simulink model "SEL751Test_Model_1"  (Simulink 8.1)
settings: Solver=ode4  StartTime=0.0  StopTime=inf  FixedStep=Ts  MaxStep=1e-3  RelTol=1e-3
PostLoadFcn:
  | Ts=100e-6; HILLTOP_init;SIM_HIL=1
InitFcn:
  | Ts=100e-6; HILLTOP_init;SIM_HIL=1
values from neighbouring files (symbols this model uses):
  relay_par = xlsread('relay_parameters.xlsx')    [relay_settings_init.m]
undefined symbols (not defined in the file or in its folder): fdesignblkfcn, gcbh, Left, NG_CHP, NG_CHP_lib, ph, type, V
libraries: simulink x23, rtio_opalrt_common x21, rtlab x7, simulink_extras x7, artemis x5, rteventslib x4, Load_lib x3, cables_lib x3, breaker_lib x3, powerlib x2, rtio_generic_modbus x2, transformer_lib x2
(part 2 of 2)

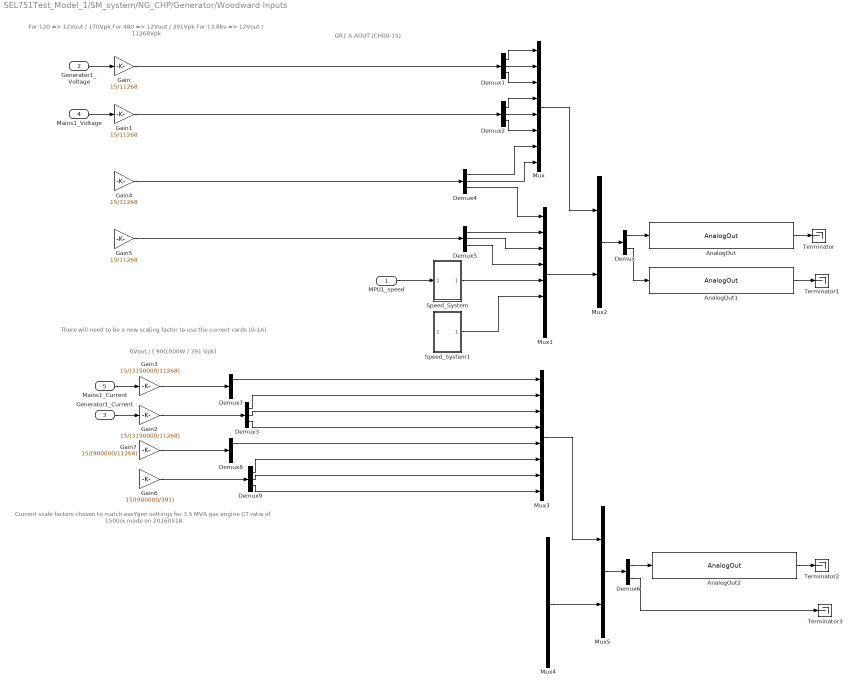
== system SEL751Test_Model_1/SM_system/NG_CHP/Generator/Woodward Inputs ==
  note: There will need to be a
      | new scaling factor to use
      | the current cards (0-1A)
  note: GR1 A AOUT (CH00-15)
  note: For 120 => 12Vout / 170Vpk
      | For 480 => 12Vout / 391Vpk
      | For 13.8kv => 12Vout / 11268Vpk
  note: 6Vout / ( 900,000W / 391 Vpk)
  note: Current scale factors chosen to match
      | easYgen settings for 3.5 MVA gas engine
      | CT ratio of 1500/x made on 20160518
  MPU1_speed : Inport
  Generator1_Voltage : Inport  Port=2
  Generator1_Current : Inport  Port=3
  Mains1_Voltage : Inport  Port=4
  Mains1_Current : Inport  Port=5
  AnalogOut : rtio_opalrt_common/AnalogOut  CtrlName='OpCtrl'  portNb=1  FcnNos=Slot 1 Module A Subsection 1  size=16  maxcount=8  count=8  numchan=8  israngeinput=off  voltagerange=[-16 ... 16]  slot=0  side=0  mismatch=0  slotside=Slot_1_Module_A
      settings: AttributesFormatString=%<CtrlName>
  AnalogOut1 : rtio_opalrt_common/AnalogOut  CtrlName='OpCtrl'  portNb=2  FcnNos=Slot 1 Module A Subsection 2  size=16  maxcount=8  count=8  numchan=8  israngeinput=off  voltagerange=[-16 ... 16]  slot=0  side=0  mismatch=0  slotside=Slot_1_Module_A
      settings: AttributesFormatString=%<CtrlName>
  AnalogOut2 : rtio_opalrt_common/AnalogOut  CtrlName='OpCtrl'  portNb=3  FcnNos=Slot 2 Module A Subsection 1  size=16  maxcount=8  count=8  numchan=8  israngeinput=off  voltagerange=[-16 ... 16]  slot=1  side=0  mismatch=0  slotside=Slot_2_Module_A
      settings: AttributesFormatString=%<CtrlName>
  Demux : Demux  Outputs=2
  Demux{1..5,7..9} (8 alike) : Demux  Outputs=3
  Demux6 : Demux  Outputs=2
  Gain{,1,4..5} (4 alike) : Gain  Gain=15/11268
  Gain2 : Gain  Gain=15/(3150000/11268)
  Gain3 : Gain  Gain=15/(3150000/11268)
  Gain6 : Gain  Gain=15/(900000/391)
  Gain7 : Gain  Gain=15/(900000/11268)
  Mux{,1,3..4} (4 alike) : Mux  Inputs=8
  Mux2 : Mux  Inputs=2
  Mux5 : Mux  Inputs=2
  Speed_System : Subsystem
  Speed_System1 : Subsystem
  Terminator{,1..3} (4 alike) : Terminator
  wires:
  Demux9/3 -> Mux3/8
  Demux9/2 -> Mux3/7
  Demux9/1 -> Mux3/6
  Gain6/1 -> Demux9/1
  Demux8/1 -> Mux3/5
  Gain7/1 -> Demux8/1
  ? -> Gain7/1
  ? -> Gain6/1
  Speed_System1/1(Out1) -> Mux1/6
  ? -> Speed_System1/1(In1)
  ? -> Gain4/1
  ? -> Gain5/1
  Gain4/1 -> Demux4/1
  Gain5/1 -> Demux5/1
  Demux7/1 -> Mux3/1
  Gain3/1 -> Demux7/1
  Mains1_Current/1 -> Gain3/1
  Demux3/3 -> Mux3/4
  Demux3/2 -> Mux3/3
  Demux3/1 -> Mux3/2
  Gain2/1 -> Demux3/1
  AnalogOut2/1 -> Terminator2/1
  Demux6/2 -> Terminator3/1
  Demux6/1 -> AnalogOut2/1
  Mux3/1 -> Mux5/1
  Mux4/1 -> Mux5/2
  Mux5/1 -> Demux6/1
  Demux5/3 -> Mux1/4
  Demux5/2 -> Mux1/3
  Demux5/1 -> Mux1/2
  Demux4/3 -> Mux1/1
  Demux4/2 -> Mux/8
  Demux4/1 -> Mux/7
  Speed_System/1(Out1) -> Mux1/5
  Demux2/3 -> Mux/6
  Demux2/2 -> Mux/5
  Demux2/1 -> Mux/4
  Demux1/3 -> Mux/3
  Demux1/2 -> Mux/2
  Demux1/1 -> Mux/1
  AnalogOut/1 -> Terminator/1
  AnalogOut1/1 -> Terminator1/1
  Demux/1 -> AnalogOut/1
  Demux/2 -> AnalogOut1/1
  Generator1_Voltage/1 -> Gain/1
  Mux/1 -> Mux2/1
  Mux1/1 -> Mux2/2
  Mux2/1 -> Demux/1
  Mains1_Voltage/1 -> Gain1/1
  Gain/1 -> Demux1/1
  Gain1/1 -> Demux2/1
  Generator1_Current/1 -> Gain2/1
  MPU1_speed/1 -> Speed_System/1(In1)

== system SEL751Test_Model_1/SM_system/NG_CHP/Generator/Woodward Outputs ==
  Digital Output : Inport
  DIO Enable : Inport  Port=2
  Bias Enable : Inport  Port=3
  Gen1 MCB Status : Inport  Port=4
  Gen2 MCB Status : Inport  Port=5
  Bus Creator1 : BusCreator  Inputs=3
  DIO - Gr3 : Subsystem
  DIO - Woodward : Subsystem
  DOUT type config : Subsystem
  OpCtrl : rtio_opalrt_common/OpCtrl  CtrlName='OpCtrl'  boardid=0  BitstreamFilename=VC707_2-EX-0001-2_2_6_61-32AIO16DIO16DIOSel-01-01.bin  numconfig=-1  mode=Master  externalClock=off  decimRtsi=0  calibIO=off  SampleTime=0  loadinport=-1  BoardType=VC707  SecondaryPresent=off  sync_type=Audio
  PWM IO - Gr3 : Subsystem
  TSDIO - Gr3 : Subsystem
  Woodward Primary Inputs : Subsystem
  Error : Outport
  IDs : Outport  Port=2
  Digital Inputs : Outport  Port=3
  Gen1 Gov and AVR : Outport  Port=4
  Gen1 Fuel Enable : Outport  Port=5
  Gen1 GCB : Outport  Port=6
  Gen1 MCB : Outport  Port=7
  wires:
  Gen2 MCB Status/1 -> DIO - Woodward/6(Gen2 MCB Status)
  Gen1 MCB Status/1 -> DIO - Woodward/5(Gen1 MCB Status)
  DIO - Woodward/1(Gen1 Fuel Enable) -> Gen1 Fuel Enable/1
  DIO - Woodward/3(Gen1 MCB) -> Gen1 MCB/1
  DIO - Woodward/2(Gen1 GCB) -> Gen1 GCB/1
  Digital Output/1 -> TSDIO - Gr3/1(TSDout), PWM IO - Gr3/1(PWMOut), DIO - Woodward/2(Din_sim)
  Bias Enable/1 -> Woodward Primary Inputs/1(Bias-ctrl)
  Woodward Primary Inputs/1(Gen1 Gov and AVR) -> Gen1 Gov and AVR/1
  DIO Enable/1 -> DIO - Woodward/4(control1), DIO - Woodward/3(control)
  Bus Creator1/1 -> Digital Inputs/1
  DIO - Gr3/1(DIn) -> DIO - Woodward/1(Din_Wood1), Bus Creator1/1  "DIN"
  TSDIO - Gr3/1(TSDin) -> Bus Creator1/2  "TSDIN"
  PWM IO - Gr3/1(PWMIn) -> Bus Creator1/3  "PWMIN"
  DIO - Woodward/4(DIn1) -> DIO - Gr3/1(Dout)
  OpCtrl/2 -> IDs/1
  OpCtrl/1 -> Error/1

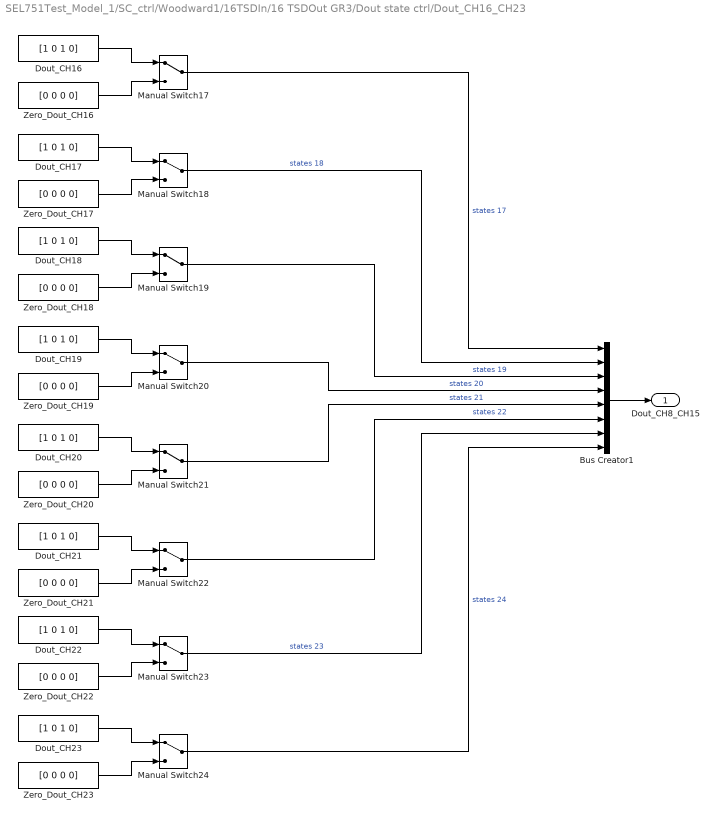
== system SEL751Test_Model_1/SC_ctrl/Woodward1/16TSDIn/16 TSDOut GR3/Dout state ctrl/Dout_CH16_CH23 ==
  Bus Creator1 : BusCreator  Inputs=8
  Dout_CH{16..23} (8 alike) : Constant  Value=[1 0 1 0]
  Manual Switch{17..24} (8 alike) : ManualSwitch
  Zero_Dout_CH{16..23} (8 alike) : Constant  Value=[0 0 0 0]
  Dout_CH8_CH15 : Outport
  wires:
  Bus Creator1/1 -> Dout_CH8_CH15/1
  Dout_CH16/1 -> Manual Switch17/1
  Zero_Dout_CH16/1 -> Manual Switch17/2
  Dout_CH17/1 -> Manual Switch18/1
  Zero_Dout_CH17/1 -> Manual Switch18/2
  Dout_CH18/1 -> Manual Switch19/1
  Zero_Dout_CH18/1 -> Manual Switch19/2
  Dout_CH19/1 -> Manual Switch20/1
  Zero_Dout_CH19/1 -> Manual Switch20/2
  Dout_CH20/1 -> Manual Switch21/1
  Zero_Dout_CH20/1 -> Manual Switch21/2
  Dout_CH21/1 -> Manual Switch22/1
  Zero_Dout_CH21/1 -> Manual Switch22/2
  Dout_CH22/1 -> Manual Switch23/1
  Zero_Dout_CH22/1 -> Manual Switch23/2
  Dout_CH23/1 -> Manual Switch24/1
  Zero_Dout_CH23/1 -> Manual Switch24/2
  Manual Switch17/1 -> Bus Creator1/1  "states 17"
  Manual Switch18/1 -> Bus Creator1/2  "states 18"
  Manual Switch19/1 -> Bus Creator1/3  "states 19"
  Manual Switch20/1 -> Bus Creator1/4  "states 20"
  Manual Switch21/1 -> Bus Creator1/5  "states 21"
  Manual Switch22/1 -> Bus Creator1/6  "states 22"
  Manual Switch23/1 -> Bus Creator1/7  "states 23"
  Manual Switch24/1 -> Bus Creator1/8  "states 24"

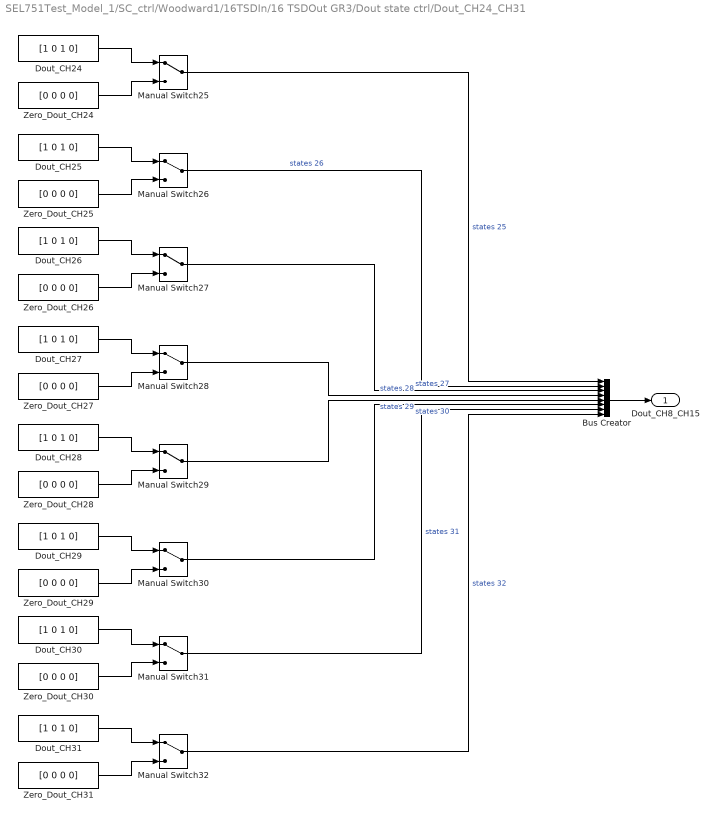
== system SEL751Test_Model_1/SC_ctrl/Woodward1/16TSDIn/16 TSDOut GR3/Dout state ctrl/Dout_CH24_CH31 ==
  Bus Creator : BusCreator  Inputs=8
  Dout_CH{24..31} (8 alike) : Constant  Value=[1 0 1 0]
  Manual Switch{25..32} (8 alike) : ManualSwitch
  Zero_Dout_CH{24..31} (8 alike) : Constant  Value=[0 0 0 0]
  Dout_CH8_CH15 : Outport
  wires:
  Manual Switch32/1 -> Bus Creator/8  "states 32"
  Manual Switch31/1 -> Bus Creator/7  "states 31"
  Manual Switch30/1 -> Bus Creator/6  "states 30"
  Manual Switch29/1 -> Bus Creator/5  "states 29"
  Manual Switch28/1 -> Bus Creator/4  "states 28"
  Manual Switch27/1 -> Bus Creator/3  "states 27"
  Manual Switch26/1 -> Bus Creator/2  "states 26"
  Manual Switch25/1 -> Bus Creator/1  "states 25"
  Zero_Dout_CH31/1 -> Manual Switch32/2
  Dout_CH31/1 -> Manual Switch32/1
  Zero_Dout_CH30/1 -> Manual Switch31/2
  Dout_CH30/1 -> Manual Switch31/1
  Zero_Dout_CH29/1 -> Manual Switch30/2
  Dout_CH29/1 -> Manual Switch30/1
  Zero_Dout_CH28/1 -> Manual Switch29/2
  Dout_CH28/1 -> Manual Switch29/1
  Zero_Dout_CH27/1 -> Manual Switch28/2
  Dout_CH27/1 -> Manual Switch28/1
  Zero_Dout_CH26/1 -> Manual Switch27/2
  Dout_CH26/1 -> Manual Switch27/1
  Zero_Dout_CH25/1 -> Manual Switch26/2
  Dout_CH25/1 -> Manual Switch26/1
  Zero_Dout_CH24/1 -> Manual Switch25/2
  Dout_CH24/1 -> Manual Switch25/1
  Bus Creator/1 -> Dout_CH8_CH15/1

== system SEL751Test_Model_1/SM_system/NG_CHP/Generator/Woodward Inputs/Speed_System ==
  In1 : Inport
  Clock1 : Clock
      settings: DisableCoverage=on
  Duty : Constant  DisableCoverage=on  Value=0.5
  Gain1 : Gain  Gain=5
  Gain3 : Gain  Gain=5
  Gain4 : Gain  Gain=1800
  Output : Trigonometry
  Product1 : Product  DisableCoverage=on  SaturateOnIntegerOverflow=on  InputSameDT=on  OutDataTypeStr=Inherit: Same as first input
  Product3 : Product  DisableCoverage=on  SaturateOnIntegerOverflow=on  InputSameDT=on  OutDataTypeStr=Inherit: Same as first input
  RTE Conversion : rteventslib/Signal Attributes/RTE Conversion  inputdatatype=RTE Boolean  outputdatatype=Double  compensation=Disabled  nbMaxEvents=10  sampleTime=Ts
  RTE SPWM : rteventslib/Sources/RTE SPWM  NumberPhases=1-ph  CenterAlignmentMode=On  MaxFreq=inf  MinFreq=0  EnablingPort=off  ComplementaryMode=off  SpaceVector=off  RiseTimeDelay=0  MaxEvents=10  SampleTime=Ts
  initialFreq : Constant  DisableCoverage=on  Value=2*pi
  Out1 : Outport
  wires:
  Product1/1 -> Output/1
  Clock1/1 -> Product1/1
  initialFreq/1 -> Product3/1
  Product3/1 -> Product1/2
  Gain4/1 -> Product3/2, RTE SPWM/1
  Output/1 -> Gain3/1
  In1/1 -> Gain4/1
  RTE SPWM/1 -> RTE Conversion/1
  Duty/1 -> RTE SPWM/2
  RTE Conversion/1 -> Gain1/1
  Gain1/1 -> Out1/1

== system SEL751Test_Model_1/SM_system/NG_CHP/Generator/Woodward Inputs/Speed_System1 ==
  In1 : Inport
  Clock1 : Clock
      settings: DisableCoverage=on
  Duty : Constant  DisableCoverage=on  Value=0.5
  Gain1 : Gain  Gain=5
  Gain3 : Gain  Gain=5
  Gain4 : Gain  Gain=1800
  Output : Trigonometry
  Product1 : Product  DisableCoverage=on  SaturateOnIntegerOverflow=on  InputSameDT=on  OutDataTypeStr=Inherit: Same as first input
  Product3 : Product  DisableCoverage=on  SaturateOnIntegerOverflow=on  InputSameDT=on  OutDataTypeStr=Inherit: Same as first input
  RTE Conversion : rteventslib/Signal Attributes/RTE Conversion  inputdatatype=RTE Boolean  outputdatatype=Double  compensation=Disabled  nbMaxEvents=10  sampleTime=Ts
  RTE SPWM : rteventslib/Sources/RTE SPWM  NumberPhases=1-ph  CenterAlignmentMode=On  MaxFreq=inf  MinFreq=0  EnablingPort=off  ComplementaryMode=off  SpaceVector=off  RiseTimeDelay=0  MaxEvents=10  SampleTime=Ts
  initialFreq : Constant  DisableCoverage=on  Value=2*pi
  Out1 : Outport
  wires:
  Product1/1 -> Output/1
  Clock1/1 -> Product1/1
  initialFreq/1 -> Product3/1
  Product3/1 -> Product1/2
  Gain4/1 -> Product3/2, RTE SPWM/1
  Output/1 -> Gain3/1
  In1/1 -> Gain4/1
  RTE SPWM/1 -> RTE Conversion/1
  Duty/1 -> RTE SPWM/2
  RTE Conversion/1 -> Gain1/1
  Gain1/1 -> Out1/1

== system SEL751Test_Model_1/SM_system/NG_CHP/Generator/Woodward Outputs/DIO - Gr3 ==
  Dout : Inport
  Bus Creator : BusCreator  Inputs=2
  Bus Selector : BusSelector  OutputSignals=DI_CH00-07  OutputAsBus=on
  Bus Selector1 : BusSelector  OutputSignals=DI_CH08-15  OutputAsBus=on
  Conditioning : Subsystem
  Conditioning1 : Subsystem
  DigitalIn : rtio_opalrt_common/DigitalIn  CtrlName='OpCtrl'  portNb=5  FcnNos=Slot 3 Module A Subsection 1  size=1  maxcount=8  count=8  sampleTime=0  numchan=8
      settings: AttributesFormatString=%<CtrlName>
  DigitalOut : rtio_opalrt_common/DigitalOut  CtrlName='OpCtrl'  portNb=5  FcnNos=Slot 3 Module B Subsection 1  size=1  maxcount=8  count=8  numchan=8
      settings: AttributesFormatString=%<CtrlName>
  Terminator1 : Terminator
  Terminator3 : Terminator
  Terminator5 : Terminator
  DIn : Outport
  wires:
  Conditioning1/1(Out1) -> Bus Creator/2
  Conditioning/1(Out1) -> Bus Creator/1
  Bus Creator/1 -> DIn/1
  DigitalIn/1 -> Conditioning/1(In1)  "DI_CH00-07"
  DigitalIn/2 -> Terminator5/1
  Bus Selector/1 -> DigitalOut/1
  Dout/1 -> Bus Selector1/1, Bus Selector/1
  Bus Selector1/1 -> Terminator1/1
  DigitalOut/1 -> Terminator3/1

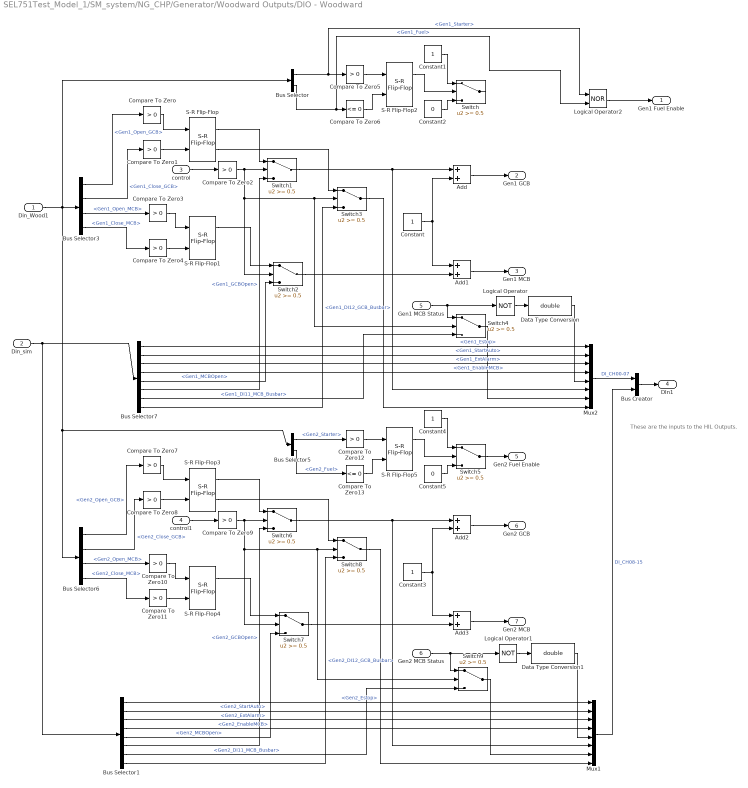
== system SEL751Test_Model_1/SM_system/NG_CHP/Generator/Woodward Outputs/DIO - Woodward ==
  note: These are the inputs to
      | the HIL Outputs.
  Din_Wood1 : Inport
  Din_sim : Inport  Port=2
  control : Inport  Port=3
  control1 : Inport  Port=4
  Gen1 MCB Status : Inport  Port=5
  Gen2 MCB Status : Inport  Port=6
  Add{,1..3} (4 alike) : Sum
  Bus Creator : BusCreator  Inputs=2
  Bus Selector : BusSelector  OutputSignals=DI_CH00-07.Gen1_Starter,DI_CH00-07.Gen1_Fuel
  Bus Selector1 : BusSelector  OutputSignals=16 DOUT GR3.08-11.Gen2_Estop,16 DOUT GR3.08-11.Gen2_StartAuto,16 DOUT GR3.08-11.Gen2_ExtAlarm,16 DOUT GR3.08-11.Gen2_EnableMCB,16 DOUT GR3.12-15.Gen2_MCBOpen,16 DOUT GR3.12-15.Gen2_GCBOpen,16 DOUT GR3.12-15.Gen2_DI11_MCB_Busbar,16 DOUT GR3.12-15.Gen2_DI12_GCB_Busbar
  Bus Selector3 : BusSelector  OutputSignals=DI_CH00-07.Gen1_Open_GCB,DI_CH00-07.Gen1_Close_GCB,DI_CH00-07.Gen1_Open_MCB,DI_CH00-07.Gen1_Close_MCB
  Bus Selector5 : BusSelector  OutputSignals=DI_CH08-15.Gen2_Starter,DI_CH08-15.Gen2_Fuel
  Bus Selector6 : BusSelector  OutputSignals=DI_CH08-15.Gen2_Open_GCB,DI_CH08-15.Gen2_Close_GCB,DI_CH08-15.Gen2_Open_MCB,DI_CH08-15.Gen2_Close_MCB
  Bus Selector7 : BusSelector  OutputSignals=16 DOUT GR3.00-03.Gen1_Estop,16 DOUT GR3.00-03.Gen1_StartAuto,16 DOUT GR3.00-03.Gen1_ExtAlarm,16 DOUT GR3.00-03.Gen1_EnableMCB,16 DOUT GR3.04-07.Gen1_MCBOpen,16 DOUT GR3.04-07.Gen1_GCBOpen,16 DOUT GR3.04-07.Gen1_DI11_MCB_Busbar,16 DOUT GR3.04-07.Gen1_DI12_GCB_Busbar
  Compare To Zero{,1..5,7..12} (12 alike) : simulink/Logic and Bit Operations/Compare To Zero  relop=>  OutDataTypeStr=boolean
  Compare To Zero13 : simulink/Logic and Bit Operations/Compare To Zero  relop=<=  OutDataTypeStr=boolean
  Compare To Zero6 : simulink/Logic and Bit Operations/Compare To Zero  relop=<=  OutDataTypeStr=boolean
  Constant{,1,3..4} (4 alike) : Constant
  Constant2 : Constant  Value=0
  Constant5 : Constant  Value=0
  Data Type Conversion : DataTypeConversion  OutDataTypeStr=double
  Data Type Conversion1 : DataTypeConversion  OutDataTypeStr=double
  Logical Operator : Logic  Operator=NOT  AllPortsSameDT=off  OutDataTypeStr=boolean
  Logical Operator1 : Logic  Operator=NOT  AllPortsSameDT=off  OutDataTypeStr=boolean
  Logical Operator2 : Logic  Operator=NOR  AllPortsSameDT=off  OutDataTypeStr=boolean
  Mux1 : Mux  Inputs=8
  Mux2 : Mux  Inputs=8
  S-R Flip-Flop{,1,3..4} (4 alike) : simulink_extras/Flip Flops/S-R Flip-Flop  initial_condition=1
  S-R Flip-Flop2 : simulink_extras/Flip Flops/S-R Flip-Flop  initial_condition=0
  S-R Flip-Flop5 : simulink_extras/Flip Flops/S-R Flip-Flop  initial_condition=0
  Switch : Switch  Threshold=0.5
  Switch{1..4,6..9} (8 alike) : Switch  Threshold=0.5  OutDataTypeStr=double
      Switch8 settings: LockScale=on
  Switch5 : Switch  Threshold=0.5
  Gen1 Fuel Enable : Outport
  Gen1 GCB : Outport  Port=2
  Gen1 MCB : Outport  Port=3
  DIn1 : Outport  Port=4
  Gen2 Fuel Enable : Outport  Port=5
  Gen2 GCB : Outport  Port=6
  Gen2 MCB : Outport  Port=7
  wires:
  Logical Operator2/1 -> Gen1 Fuel Enable/1
  Data Type Conversion1/1 -> Mux1/5
  Logical Operator1/1 -> Data Type Conversion1/1
  Gen2 MCB Status/1 -> Switch9/1, Logical Operator1/1
  Logical Operator/1 -> Data Type Conversion/1
  Data Type Conversion/1 -> Mux2/5
  Gen1 MCB Status/1 -> Switch4/1, Logical Operator/1
  Switch8/1 -> Mux1/8
  Bus Selector1/8 -> Switch8/3  "<Gen2_DI12_GCB_Busbar>"
  Switch9/1 -> Mux1/7
  Bus Selector1/7 -> Switch9/3  "<Gen2_DI11_MCB_Busbar>"
  Switch3/1 -> Mux2/8
  Bus Selector7/8 -> Switch3/3  "<Gen1_DI12_GCB_Busbar>"
  Switch4/1 -> Mux2/7
  Bus Selector7/7 -> Switch4/3  "<Gen1_DI11_MCB_Busbar>"
  Din_sim/1 -> Bus Selector1/1, Bus Selector7/1
  Mux2/1 -> Bus Creator/1  "DI_CH00-07"
  Bus Selector7/6 -> Switch1/3  "<Gen1_GCBOpen>"
  Bus Selector7/5 -> Switch2/3  "<Gen1_MCBOpen>"
  Bus Selector7/4 -> Mux2/4  "<Gen1_EnableMCB>"
  Bus Selector7/3 -> Mux2/3  "<Gen1_ExtAlarm>"
  Bus Selector7/2 -> Mux2/2  "<Gen1_StartAuto>"
  Bus Selector7/1 -> Mux2/1  "<Gen1_Estop>"
  Bus Selector1/6 -> Switch6/3  "<Gen2_GCBOpen>"
  Bus Selector1/5 -> Switch7/3  "<Gen2_MCBOpen>"
  Bus Selector1/4 -> Mux1/4  "<Gen2_EnableMCB>"
  Bus Selector1/3 -> Mux1/3  "<Gen2_ExtAlarm>"
  Bus Selector1/2 -> Mux1/2  "<Gen2_StartAuto>"
  Bus Selector1/1 -> Mux1/1  "<Gen2_Estop>"
  Bus Selector3/3 -> Compare To Zero3/1  "<Gen1_Open_MCB>"
  Switch5/1 -> Gen2 Fuel Enable/1
  Compare To Zero13/1 -> S-R Flip-Flop5/2
  Constant4/1 -> Switch5/1
  Constant5/1 -> Switch5/3
  Compare To Zero12/1 -> S-R Flip-Flop5/1
  S-R Flip-Flop5/1 -> Switch5/2
  Bus Selector5/2 -> Compare To Zero13/1  "<Gen2_Fuel>"
  Bus Selector5/1 -> Compare To Zero12/1  "<Gen2_Starter>"
  Constant3/1 -> Add3/1, Add2/2
  Add3/1 -> Gen2 MCB/1
  Add2/1 -> Gen2 GCB/1
  S-R Flip-Flop3/2 -> Switch8/1
  Switch7/1 -> Add3/2
  Compare To Zero9/1 -> Switch9/2, Switch8/2, Switch7/2, Switch6/2
  Bus Selector6/2 -> Compare To Zero8/1  "<Gen2_Close_GCB>"
  S-R Flip-Flop4/1 -> Switch7/1
  Compare To Zero10/1 -> S-R Flip-Flop4/1
  Bus Selector6/3 -> Compare To Zero10/1  "<Gen2_Open_MCB>"
  Compare To Zero11/1 -> S-R Flip-Flop4/2
  Bus Selector6/4 -> Compare To Zero11/1  "<Gen2_Close_MCB>"
  Compare To Zero8/1 -> S-R Flip-Flop3/2
  Compare To Zero7/1 -> S-R Flip-Flop3/1
  Bus Selector6/1 -> Compare To Zero7/1  "<Gen2_Open_GCB>"
  Switch6/1 -> Mux1/6, Add2/1
  S-R Flip-Flop3/1 -> Switch6/1
  control1/1 -> Compare To Zero9/1
  Compare To Zero6/1 -> S-R Flip-Flop2/2
  Constant1/1 -> Switch/1
  Constant2/1 -> Switch/3
  Compare To Zero5/1 -> S-R Flip-Flop2/1
  S-R Flip-Flop2/1 -> Switch/2
  Bus Selector/2 -> Compare To Zero6/1, Logical Operator2/2  "<Gen1_Fuel>"
  Bus Selector/1 -> Compare To Zero5/1, Logical Operator2/1  "<Gen1_Starter>"
  Constant/1 -> Add1/1, Add/2
  Add1/1 -> Gen1 MCB/1
  Add/1 -> Gen1 GCB/1
  S-R Flip-Flop/2 -> Switch3/1
  Mux1/1 -> Bus Creator/2  "DI_CH08-15"
  Switch2/1 -> Add1/2
  Compare To Zero2/1 -> Switch4/2, Switch3/2, Switch2/2, Switch1/2
  S-R Flip-Flop1/1 -> Switch2/1
  Compare To Zero3/1 -> S-R Flip-Flop1/1
  Compare To Zero4/1 -> S-R Flip-Flop1/2
  Bus Selector3/4 -> Compare To Zero4/1  "<Gen1_Close_MCB>"
  Compare To Zero1/1 -> S-R Flip-Flop/2
  Compare To Zero/1 -> S-R Flip-Flop/1
  Switch1/1 -> Mux2/6, Add/1
  S-R Flip-Flop/1 -> Switch1/1
  Bus Creator/1 -> DIn1/1
  control/1 -> Compare To Zero2/1
  Din_Wood1/1 -> Bus Selector5/1, Bus Selector6/1, Bus Selector/1, Bus Selector3/1
  Bus Selector3/1 -> Compare To Zero/1  "<Gen1_Open_GCB>"
  Bus Selector3/2 -> Compare To Zero1/1  "<Gen1_Close_GCB>"

== system SEL751Test_Model_1/SM_system/NG_CHP/Generator/Woodward Outputs/DOUT type config ==
  note: The Constants are used to select Digital Output type:
      | - 0: Time-Stamped Digital Output
      | - 1: Pulse-Width Modulated DIgital Output
  DataIn Send : rtio_opalrt_common/DataIn Send  CtrlName='OpCtrl'  FcnNos=11  width=1  portType=double  checkVersion=off  expectedId=0  expectedVersion=0  opComp=>=
      settings: AttributesFormatString=%<CtrlName>
  DataIn Send1 : rtio_opalrt_common/DataIn Send  CtrlName='OpCtrl'  FcnNos=12  width=1  portType=double  checkVersion=off  expectedId=0  expectedVersion=0  opComp=>=
      settings: AttributesFormatString=%<CtrlName>
  Subsection 3 DOUT type : Constant
  Subsection 4 DOUT type : Constant
  Terminator1 : Terminator
  Terminator2 : Terminator
  wires:
  DataIn Send/1 -> Terminator2/1
  DataIn Send1/1 -> Terminator1/1
  Subsection 4 DOUT type/1 -> DataIn Send1/1
  Subsection 3 DOUT type/1 -> DataIn Send/1

== system SEL751Test_Model_1/SM_system/NG_CHP/Generator/Woodward Outputs/PWM IO - Gr3 ==
  PWMOut : Inport
  Bus Creator : BusCreator  Inputs=2
  Bus Creator1 : BusCreator  Inputs=2
  Bus Creator2 : BusCreator  Inputs=2
  Bus Selector : BusSelector  OutputSignals=FreqPWMOut16-23,DutyPWMOut16-23
  Bus Selector1 : BusSelector  OutputSignals=FreqPWMOut24-31,DutyPWMOut24-31
  Bus Selector2 : BusSelector  OutputSignals=16 PWMOUT GR3.Ch16-23,16 PWMOUT GR3.Ch24-31
  PWM In : rtio_opalrt_common/PWM In  CtrlName='OpCtrl'  portNb=9  FcnNos=Slot 3 Module A Subsection 3  maxCount=8  Count=8  sampleTime=0  numchan=8
      settings: AttributesFormatString=%<CtrlName>
  PWM In1 : rtio_opalrt_common/PWM In  CtrlName='OpCtrl'  portNb=10  FcnNos=Slot 3 Module A Subsection 4  maxCount=8  Count=8  sampleTime=0  numchan=8
      settings: AttributesFormatString=%<CtrlName>
  PWM Out : rtio_opalrt_common/PWM Out  CtrlName='OpCtrl'  portNb=9  FcnNos=Slot 3 Module B Subsection 3  size=64  maxcount=8  count=8  polarity=Active High  symMode=Symmetric  complementary=off  deadTime=0  numchan=8  loadnb=1  initphase=[0 0 0 0 0 0 0 0]
      settings: AttributesFormatString=%<CtrlName>
  PWM Out1 : rtio_opalrt_common/PWM Out  CtrlName='OpCtrl'  portNb=10  FcnNos=Slot 3 Module B Subsection 4  size=64  maxcount=8  count=8  polarity=Active High  symMode=Symmetric  complementary=off  deadTime=0  numchan=8  loadnb=2  initphase=[0 0 0 0 0 0 0 0]
      settings: AttributesFormatString=%<CtrlName>
  Terminator{,1,4..5} (4 alike) : Terminator
  PWMIn : Outport
  wires:
  Bus Selector2/2 -> Bus Selector1/1  "<Ch24-31>"
  PWM In1/2 -> Bus Creator2/2  "Duty"
  PWM In1/1 -> Bus Creator2/1  "Freq"
  PWM In/2 -> Bus Creator1/2  "Duty"
  PWM In/1 -> Bus Creator1/1  "Freq"
  PWM In/3 -> Terminator4/1
  PWM In1/3 -> Terminator5/1
  Bus Creator2/1 -> Bus Creator/2  "PWMI_CH24-31"
  Bus Creator1/1 -> Bus Creator/1  "PWMI_CH16-23"
  Bus Creator/1 -> PWMIn/1
  Bus Selector2/1 -> Bus Selector/1  "<Ch16-23>"
  PWMOut/1 -> Bus Selector2/1
  PWM Out1/1 -> Terminator1/1
  Bus Selector1/2 -> PWM Out1/2  "<DutyPWMOut24-31>"
  Bus Selector1/1 -> PWM Out1/1  "<FreqPWMOut24-31>"
  PWM Out/1 -> Terminator/1
  Bus Selector/2 -> PWM Out/2  "<DutyPWMOut16-23>"
  Bus Selector/1 -> PWM Out/1  "<FreqPWMOut16-23>"

== system SEL751Test_Model_1/SM_system/NG_CHP/Generator/Woodward Outputs/TSDIO - Gr3 ==
  TSDout : Inport
  Bus Creator : BusCreator  Inputs=16
  Bus Creator1 : BusCreator  Inputs=16
  Bus Creator2 : BusCreator  Inputs=2
  Bus Selector : BusSelector  OutputSignals=16 TSDOUT GR3.states.CH16-23.states 17,16 TSDOUT GR3.times CH16-23.times17,16 TSDOUT GR3.states.CH16-23.states 18,16 TSDOUT GR3.times CH16-23.times18,16 TSDOUT GR3.states.CH16-23.states 19,16 TSDOUT GR3.times CH16-23.times19,16 TSDOUT GR3.states.CH16-23.states 20,16 TSDOUT GR3.times CH16-23.times20,16 TSDOUT GR3.states.CH16-23.states 21,16 TSDOUT GR3.times CH16-23.times21,16 TSDOUT GR3.states.CH16-23.states 22,16 TSDOUT GR3.times CH16-23.times22,16 TSDOUT GR3.states.CH16-23.states 23,16 TSDOUT GR3.times CH16-23.times23,16 TSDOUT GR3.states.CH16-23.states 24,16 TSDOUT GR3.times CH16-23.times24
  Bus Selector1 : BusSelector  OutputSignals=16 TSDOUT GR3.states.CH24-31.states 25,16 TSDOUT GR3.times CH24-31.times25,16 TSDOUT GR3.states.CH24-31.states 26,16 TSDOUT GR3.times CH24-31.times26,16 TSDOUT GR3.states.CH24-31.states 27,16 TSDOUT GR3.times CH24-31.times27,16 TSDOUT GR3.states.CH24-31.states 28,16 TSDOUT GR3.times CH24-31.times28,16 TSDOUT GR3.states.CH24-31.states 29,16 TSDOUT GR3.times CH24-31.times29,16 TSDOUT GR3.states.CH24-31.states 30,16 TSDOUT GR3.times CH24-31.times30,16 TSDOUT GR3.states.CH24-31.states 31,16 TSDOUT GR3.times CH24-31.times31,16 TSDOUT GR3.states.CH24-31.states 32,16 TSDOUT GR3.times CH24-31.times32
  EventDetector : rtio_opalrt_common/EventDetector  CtrlName='OpCtrl'  portNb=7  FcnNos=Slot 3 Module A Subsection 3  size=32  maxcount=8  nbChannels=8  width=4  timeUnit=Time ratio  sampleTime=0  numwidth=4
      settings: AttributesFormatString=%<CtrlName>
  EventDetector1 : rtio_opalrt_common/EventDetector  CtrlName='OpCtrl'  portNb=8  FcnNos=Slot 3 Module A Subsection 4  size=32  maxcount=8  nbChannels=8  width=4  timeUnit=Time ratio  sampleTime=0  numwidth=4
      settings: AttributesFormatString=%<CtrlName>
  EventGenerator : rtio_opalrt_common/EventGenerator  CtrlName='OpCtrl'  portNb=7  FcnNos=Slot 3 Module B Subsection 3  size=32  count=8  nbChannels=8  width=4  timeUnit=Time ratio  numwidth=4
      settings: AttributesFormatString=%<CtrlName>
  EventGenerator1 : rtio_opalrt_common/EventGenerator  CtrlName='OpCtrl'  portNb=8  FcnNos=Slot 3 Module B Subsection 4  size=32  count=8  nbChannels=8  width=4  timeUnit=Time ratio  numwidth=4
      settings: AttributesFormatString=%<CtrlName>
  Terminator{,1..3} (4 alike) : Terminator
  TSDin : Outport
  wires:
  Bus Creator2/1 -> TSDin/1  "TSDIN"
  Bus Creator/1 -> Bus Creator2/1  "CH16-23"
  EventDetector1/17 -> Terminator3/1  "states7"
  EventDetector1/1 -> Bus Creator1/1  "states1"
  EventDetector1/2 -> Bus Creator1/2  "times1"
  EventDetector1/3 -> Bus Creator1/3  "states2"
  EventDetector1/4 -> Bus Creator1/4  "times2"
  EventDetector1/5 -> Bus Creator1/5  "states1"
  EventDetector1/6 -> Bus Creator1/6  "times1"
  EventDetector1/7 -> Bus Creator1/7  "states2"
  EventDetector1/8 -> Bus Creator1/8  "times2"
  EventDetector1/9 -> Bus Creator1/9  "states3"
  EventDetector1/10 -> Bus Creator1/10  "times3"
  EventDetector1/11 -> Bus Creator1/11  "states4"
  EventDetector1/12 -> Bus Creator1/12  "times4"
  EventDetector1/13 -> Bus Creator1/13  "states5"
  EventDetector1/14 -> Bus Creator1/14  "times5"
  EventDetector1/15 -> Bus Creator1/15  "states6"
  EventDetector1/16 -> Bus Creator1/16  "times6"
  Bus Creator1/1 -> Bus Creator2/2  "CH24-31"
  Bus Selector1/16 -> EventGenerator1/16  "<times32>"
  Bus Selector1/15 -> EventGenerator1/15  "<states 32>"
  Bus Selector1/14 -> EventGenerator1/14  "<times31>"
  Bus Selector1/13 -> EventGenerator1/13  "<states 31>"
  Bus Selector1/12 -> EventGenerator1/12  "<times30>"
  Bus Selector1/11 -> EventGenerator1/11  "<states 30>"
  Bus Selector1/10 -> EventGenerator1/10  "<times29>"
  Bus Selector1/9 -> EventGenerator1/9  "<states 29>"
  Bus Selector1/8 -> EventGenerator1/8  "<times28>"
  Bus Selector1/7 -> EventGenerator1/7  "<states 28>"
  Bus Selector1/6 -> EventGenerator1/6  "<times27>"
  Bus Selector1/5 -> EventGenerator1/5  "<states 27>"
  Bus Selector1/4 -> EventGenerator1/4  "<times26>"
  Bus Selector1/3 -> EventGenerator1/3  "<states 26>"
  Bus Selector1/2 -> EventGenerator1/2  "<times25>"
  Bus Selector1/1 -> EventGenerator1/1  "<states 25>"
  EventGenerator1/1 -> Terminator2/1
  EventDetector/17 -> Terminator1/1
  EventDetector/1 -> Bus Creator/1  "states1"
  EventDetector/2 -> Bus Creator/2  "times1"
  EventDetector/3 -> Bus Creator/3  "states2"
  EventDetector/4 -> Bus Creator/4  "times2"
  EventDetector/5 -> Bus Creator/5  "states3"
  EventDetector/6 -> Bus Creator/6  "times3"
  EventDetector/7 -> Bus Creator/7  "states4"
  EventDetector/8 -> Bus Creator/8  "times4"
  EventDetector/9 -> Bus Creator/9  "states5"
  EventDetector/10 -> Bus Creator/10  "times5"
  EventDetector/11 -> Bus Creator/11  "states6"
  EventDetector/12 -> Bus Creator/12  "times6"
  EventDetector/13 -> Bus Creator/13  "states7"
  EventDetector/14 -> Bus Creator/14  "times7"
  EventDetector/15 -> Bus Creator/15  "states8"
  EventDetector/16 -> Bus Creator/16  "times8"
  EventGenerator/1 -> Terminator/1
  Bus Selector/1 -> EventGenerator/1  "<states 17>"
  Bus Selector/2 -> EventGenerator/2  "<times17>"
  Bus Selector/3 -> EventGenerator/3  "<states 18>"
  Bus Selector/4 -> EventGenerator/4  "<times18>"
  Bus Selector/5 -> EventGenerator/5  "<states 19>"
  Bus Selector/6 -> EventGenerator/6  "<times19>"
  Bus Selector/7 -> EventGenerator/7  "<states 20>"
  Bus Selector/8 -> EventGenerator/8  "<times20>"
  Bus Selector/9 -> EventGenerator/9  "<states 21>"
  Bus Selector/10 -> EventGenerator/10  "<times21>"
  Bus Selector/11 -> EventGenerator/11  "<states 22>"
  Bus Selector/12 -> EventGenerator/12  "<times22>"
  Bus Selector/13 -> EventGenerator/13  "<states 23>"
  Bus Selector/14 -> EventGenerator/14  "<times23>"
  Bus Selector/15 -> EventGenerator/15  "<states 24>"
  Bus Selector/16 -> EventGenerator/16  "<times24>"
  TSDout/1 -> Bus Selector1/1, Bus Selector/1

== system SEL751Test_Model_1/SM_system/NG_CHP/Generator/Woodward Outputs/Woodward Primary Inputs ==
  Bias-ctrl : Inport
  Bus Creator : BusCreator
  Constant : Constant  Value=1.00
  Constant1 : Constant  Value=0
  Constant2 : Constant  Value=20
  Constant3 : Constant  Value=0
  Constant4 : Constant  Value=0
  Constant5 : Constant  Value=1.00
  Demux1 : Demux  Outputs=16
  Divide : Product  Inputs=*/
  Divide1 : Product  Inputs=*/
  GR1 B AIN (CH00-15) : Subsystem
  Lowpass Filter : Subsystem  DialogController=fdesignblkfcn  DialogControllerArgs=DataTag2  InitFcn=fdesignblkfcn(gcbh, {'InitFcn'});  mask(Lowpass Filter){}
      mask help: Design a lowpass filter
      settings: CopyFcn=fdesignblkfcn(gcbh, {'CopyFcn'});
      mask Help: helpview(mapfilelocation('dsp'), 'dsplowpassfilter');
      mask Display: disp('Lowpass')
  Lowpass Filter1 : Subsystem  DialogController=fdesignblkfcn  DialogControllerArgs=DataTag4  InitFcn=fdesignblkfcn(gcbh, {'InitFcn'});  mask(Lowpass Filter){}
      mask help: Design a lowpass filter
      settings: CopyFcn=fdesignblkfcn(gcbh, {'CopyFcn'});
      mask Help: helpview(mapfilelocation('dsp'), 'dsplowpassfilter');
      mask Display: disp('Lowpass')
  Sum : Sum  Inputs=|+-
  Sum1 : Sum  Inputs=|+-
  Switch : Switch  Threshold=0.5
  Switch1 : Switch  Threshold=0.5
  Gen1 Gov and AVR : Outport
  wires:
  Bus Creator/1 -> Gen1 Gov and AVR/1
  Constant/1 -> Bus Creator/1  "Gen1 Ref GOV"
  Constant5/1 -> Bus Creator/2  "Gen1 Ref AVR"
  Lowpass Filter1/1(Out) -> Switch1/1
  Lowpass Filter/1(Out) -> Switch/1
  Bias-ctrl/1 -> Switch1/2, Switch/2
  Constant1/1 -> Switch1/3, Switch/3
  Sum1/1 -> Lowpass Filter1/1(In)
  Switch1/1 -> Bus Creator/4  "Gen1 AVR"
  Switch/1 -> Bus Creator/3  "Gen1 Gov"
  Sum/1 -> Lowpass Filter/1(In)
  Constant4/1 -> Sum1/2
  Constant3/1 -> Sum/2
  Divide1/1 -> Sum1/1
  Divide/1 -> Sum/1
  Constant2/1 -> Divide/2, Divide1/2
  Demux1/2 -> Divide1/1
  Demux1/1 -> Divide/1
  GR1 B AIN (CH00-15)/1(Out1) -> Demux1/1, [AINs_Gr1]

== system SEL751Test_Model_1/SM_system/NG_CHP/Generator/Woodward Outputs/DIO - Gr3/Conditioning ==
  In1 : Inport
  Bus Creator : BusCreator  Inputs=8
  Demux : Demux  Outputs=8
  Out1 : Outport
  wires:
  In1/1 -> Demux/1
  Bus Creator/1 -> Out1/1  "DI_CH00-07"
  Demux/8 -> Bus Creator/8  "Gen1_Alarm_CF"
  Demux/7 -> Bus Creator/7  "Gen1_Alarm_AB"
  Demux/6 -> Bus Creator/6  "Gen1_Open_MCB"
  Demux/5 -> Bus Creator/5  "Gen1_Close_MCB"
  Demux/4 -> Bus Creator/4  "Gen1_Open_GCB"
  Demux/3 -> Bus Creator/3  "Gen1_Close_GCB"
  Demux/2 -> Bus Creator/2  "Gen1_Fuel"
  Demux/1 -> Bus Creator/1  "Gen1_Starter"

== system SEL751Test_Model_1/SM_system/NG_CHP/Generator/Woodward Outputs/DIO - Gr3/Conditioning1 ==
  In1 : Inport
  Bus Creator : BusCreator  Inputs=8
  Demux : Demux  Outputs=8
  Out1 : Outport
  wires:
  Demux/1 -> Bus Creator/1  "Gen2_Starter"
  Demux/2 -> Bus Creator/2  "Gen2_Fuel"
  Demux/3 -> Bus Creator/3  "Gen2_Close_GCB"
  Demux/4 -> Bus Creator/4  "Gen2_Open_GCB"
  Demux/5 -> Bus Creator/5  "Gen2_Close_MCB"
  Demux/6 -> Bus Creator/6  "Gen2_Open_MCB"
  Demux/7 -> Bus Creator/7  "Gen2_Alarm_AB"
  Demux/8 -> Bus Creator/8  "Gen2_Alarm_CF"
  Bus Creator/1 -> Out1/1  "DI_CH08-15"
  In1/1 -> Demux/1

== system SEL751Test_Model_1/SM_system/NG_CHP/Generator/Woodward Outputs/Woodward Primary Inputs/GR1 B AIN (CH00-15) ==
  AnalogIn : rtio_opalrt_common/AnalogIn  CtrlName='OpCtrl'  portNb=1  FcnNos=Slot 1 Module B Subsection 1  size=16  maxcount=8  count=8  numchan=8  sampleTime=0
      settings: AttributesFormatString=%<CtrlName>
  AnalogIn1 : rtio_opalrt_common/AnalogIn  CtrlName='OpCtrl'  portNb=2  FcnNos=Slot 1 Module B Subsection 2  size=16  maxcount=8  count=8  numchan=8  sampleTime=0
      settings: AttributesFormatString=%<CtrlName>
  Mux6 : Mux  Inputs=2
  Terminator2 : Terminator
  Terminator3 : Terminator
  Out1 : Outport
  wires:
  AnalogIn/1 -> Mux6/1
  AnalogIn1/1 -> Mux6/2
  AnalogIn/2 -> Terminator2/1
  AnalogIn1/2 -> Terminator3/1
  Mux6/1 -> Out1/1

== system SEL751Test_Model_1/SM_system/NG_CHP/Generator/Woodward Outputs/Woodward Primary Inputs/Lowpass Filter ==
  In : Inport
  Generated Filter Block : DiscreteFir  Tag=BlockMethodSubSystem  Coefficients=[0.0069552863617617106 0.014587901014631248 -0.0057896483056441538 -0.056861876528372622 -0.059476680260783142 0.076118200884714562 0.29579154768342669 0.40638624201187618 0.29579154768342669 0.076118200884714562 -0.059476680260783142 -0.056861876528372622 -0.0057896483056441538 0.014587901014631248 0.0069552863617617106]  InputProcessing=Columns as channels (frame based)
  Out : Outport
  wires:
  Generated Filter Block/1 -> Out/1
  In/1 -> Generated Filter Block/1

== system SEL751Test_Model_1/SM_system/NG_CHP/Generator/Woodward Outputs/Woodward Primary Inputs/Lowpass Filter1 ==
  In : Inport
  Generated Filter Block : DiscreteFir  Tag=BlockMethodSubSystem  Coefficients=[0.0069552863617617106 0.014587901014631248 -0.0057896483056441538 -0.056861876528372622 -0.059476680260783142 0.076118200884714562 0.29579154768342669 0.40638624201187618 0.29579154768342669 0.076118200884714562 -0.059476680260783142 -0.056861876528372622 -0.0057896483056441538 0.014587901014631248 0.0069552863617617106]  InputProcessing=Columns as channels (frame based)
  Out : Outport
  wires:
  Generated Filter Block/1 -> Out/1
  In/1 -> Generated Filter Block/1
